simulink subsystem "Wind"  (R2025a)
settings: Solver=VariableStepAuto  StartTime=0.0  StopTime=10.0  RelTol=1e-3
model mask{windRating=0, maxWindSpeed=0, turbineOutput=0, frequency=0, windingRatio=0, rotorSpeed=0, windSpeed=0}
  mask prompts: windRating "Rating (kW)"; maxWindSpeed "Maximum Wind speed (m/s)"; turbineOutput "Turbine output (kW)"; frequency "Frequency (Hz)"; windingRatio "Transformer Ratio"; rotorSpeed "Rotor Speed (rpm)"; windSpeed "Wind Speed (m/s)"
libraries: fl_lib x19, ee_lib x8, nesl_utility x7
settings Model: DefaultTestHarness=Wind_Harness  Creator=skota  LastModifiedBy=skota

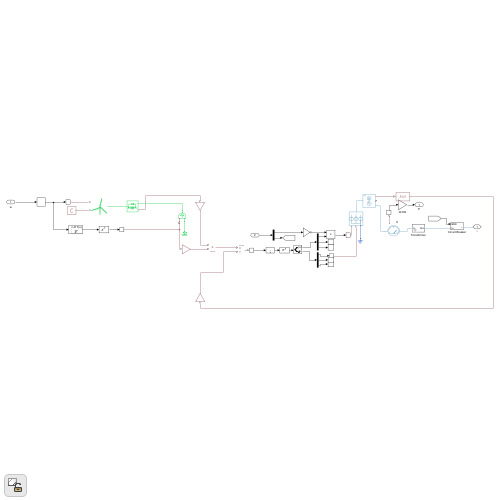
[thumbnail: Simulink's stored preview of the top-level diagram]
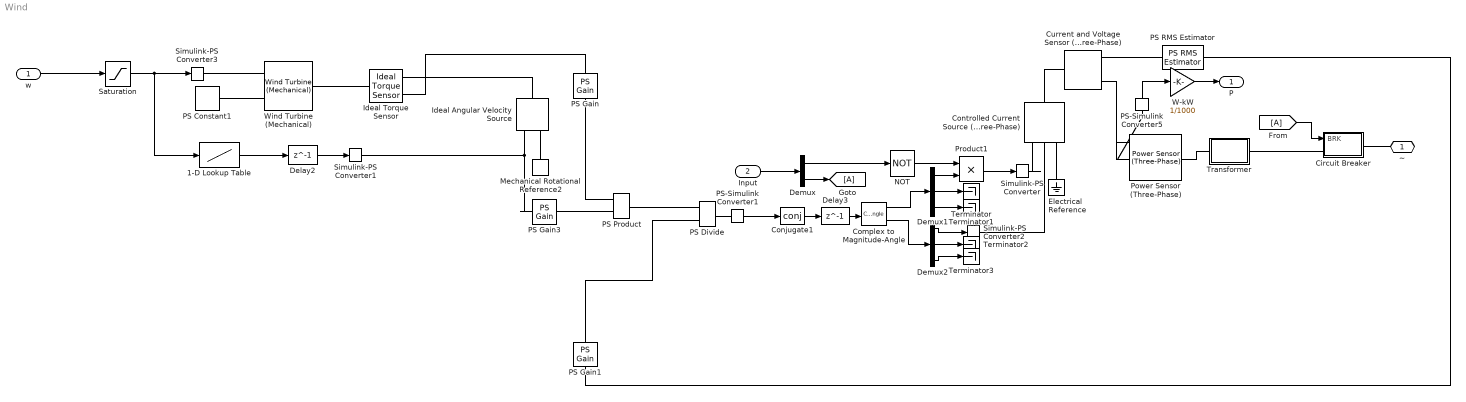
== system Wind ==
  w : Inport
  Input : Inport  Port=2
  1-D Lookup Table : Lookup_n-D  NumberOfTableDimensions=1  BreakpointsForDimension1=windSpeed  Table=rotorSpeed  InternalRulePriority=Speed  RndMeth=Simplest
  Circuit Breaker : Subsystem
  Complex to Magnitude-Angle : ComplexToMagnitudeAngle
  Conjugate1 : Math  Operator=conj  SignedPower=on  RndMeth=Zero
  Controlled Current Source (Three-Phase) : ee_lib/Sources/Controlled Current Source (Three-Phase)  input_option=ee.enum.inputType.singleFreqAC  FRated=frequency Hz
      settings: InternalSimscapePortConfiguration="{\"Bottom\":[],\"Left\":[{\"id\":\"It\",\"label\":\"I\",\"type\":\"input\"},{\"id\":\"ph\",\"label\":\"ph\",\"type\":\"input\"},{\"id\":\"n\",\"label\":\"n\",\"type\":\"foundation.electrical.electrical\"}],\"Right\":[{\"id\":\"N\",\"label\":\"~\",\"type\":\"foundation.electrical.three_phase\"}],\"Top\":[]}"
  Current and Voltage Sensor (Three-Phase) : ee_lib/Sensors & Transducers/Current and Voltage Sensor (Three-Phase)  vMeasurementType=ee.enum.vmeasurement.ll  outputUnit=ee.enum.unit.si  SRated=100e6 A*V  VRated=24e3 V  I_specify=off  I_priority=None  I=[0, 0, 0] A  I_nominal_specify=off  I_nominal_value=1  I_nominal_unit=A  V_specify=off  V_priority=None  V=[0, 0, 0] V  V_nominal_specify=off  V_nominal_value=1  V_nominal_unit=V
      settings: InternalSimscapePortConfiguration="{\"Bottom\":[],\"Left\":[{\"id\":\"N1\",\"label\":\"~1\",\"type\":\"foundation.electrical.three_phase\"}],\"Right\":[{\"id\":\"V_output\",\"label\":\"V\",\"type\":\"output\"},{\"id\":\"I_output\",\"label\":\"I\",\"type\":\"output\"},{\"id\":\"N2\",\"label\":\"~2\",\"type\":\"foundation.electrical.three_phase\"}],\"Top\":[]}"
  Delay2 : Delay  DelayLength=1  InitialCondition=1
  Delay3 : Delay  DelayLength=1  InitialCondition=1
  Demux : Demux  Outputs=2
  Demux1 : Demux  Outputs=3
  Demux2 : Demux  Outputs=3
  Electrical Reference : fl_lib/Electrical/Electrical Elements/Electrical Reference
  From : From
  Goto : Goto
  Ideal Angular Velocity Source : fl_lib/Mechanical/Mechanical Sources/Ideal Angular Velocity Source
  Ideal Torque Sensor : fl_lib/Mechanical/Mechanical Sensors/Ideal Torque Sensor
  Mechanical Rotational Reference2 : fl_lib/Mechanical/Rotational Elements/Mechanical Rotational Reference
  NOT : Logic  Operator=NOT  IconShape=distinctive  AllPortsSameDT=off  OutDataTypeStr=boolean
  PS Constant1 : fl_lib/Physical Signals/Sources/PS Constant  constant=0
  PS Divide : fl_lib/Physical Signals/Functions/PS Divide
  PS Gain : fl_lib/Physical Signals/Functions/PS Gain  gain=round(windRating/turbineOutput)
  PS Gain1 : fl_lib/Physical Signals/Functions/PS Gain  gain=sqrt(3)
  PS Gain3 : fl_lib/Physical Signals/Functions/PS Gain  gain=pi/30 rad/s
  PS Product : fl_lib/Physical Signals/Functions/PS Product
  PS RMS Estimator : fl_lib/Physical Signals/Periodic Operators/PS RMS Estimator  f0=frequency Hz
      settings: InternalSimscapePortConfiguration="{\"Bottom\":[],\"Left\":[{\"id\":\"I\",\"label\":\"\",\"type\":\"input\"}],\"Right\":[{\"id\":\"O\",\"label\":\"\",\"type\":\"output\"}],\"Top\":[]}"
  PS-Simulink Converter1 : nesl_utility/PS-Simulink Converter  PhysicalDomain=network_engine_domain  SubClassName=ps_output  LeftPortType=input  RightPortType=output  PseudoPeriodic=off  Frequencies=[]  VectorFormat=inherit  Unit=inherit  AffineConversion=off
  PS-Simulink Converter5 : nesl_utility/PS-Simulink Converter  PhysicalDomain=network_engine_domain  SubClassName=ps_output  LeftPortType=input  RightPortType=output  PseudoPeriodic=off  Frequencies=[]  VectorFormat=inherit  Unit=inherit  AffineConversion=off
  Power Sensor (Three-Phase) : ee_lib/Sensors & Transducers/Power Sensor (Three-Phase)  load_type=ee.enum.passive.type_balanced.balanced  f0=60 Hz  config=ee.enum.with_neutral.no  rho=1
      settings: InternalSimscapePortConfiguration="{\"Bottom\":[],\"Left\":[{\"id\":\"N1\",\"label\":\"~1\",\"type\":\"foundation.electrical.three_phase\"}],\"Right\":[{\"id\":\"N2\",\"label\":\"~2\",\"type\":\"foundation.electrical.three_phase\"}],\"Top\":[{\"id\":\"Pm\",\"label\":\"P\",\"type\":\"output\"},{\"id\":\"Qm\",\"label\":\"Q\",\"type\":\"output\"}]}"
  Product1 : Product
  Saturation : Saturate  UpperLimit=maxWindSpeed  LowerLimit=0
  Simulink-PS Converter : nesl_utility/Simulink-PS Converter  PhysicalDomain=network_engine_domain  SubClassName=ps_input  LeftPortType=input  RightPortType=output  PseudoPeriodic=off  Frequencies=[]  NoiseDistribution=none  NoiseParameters=[]  Unit=1  AffineConversion=off  FilteringAndDerivatives=provide  SimscapeFilterOrder=1  InputFilterTimeConstant=0.001  UdotUserProvided=0
  Simulink-PS Converter1 : nesl_utility/Simulink-PS Converter  PhysicalDomain=network_engine_domain  SubClassName=ps_input  LeftPortType=input  RightPortType=output  PseudoPeriodic=off  Frequencies=[]  NoiseDistribution=none  NoiseParameters=[]  Unit=rpm  AffineConversion=off  FilteringAndDerivatives=provide  SimscapeFilterOrder=1  InputFilterTimeConstant=0.001  UdotUserProvided=0
  Simulink-PS Converter2 : nesl_utility/Simulink-PS Converter  PhysicalDomain=network_engine_domain  SubClassName=ps_input  LeftPortType=input  RightPortType=output  PseudoPeriodic=off  Frequencies=[]  NoiseDistribution=none  NoiseParameters=[]  Unit=1  AffineConversion=off  FilteringAndDerivatives=provide  SimscapeFilterOrder=1  InputFilterTimeConstant=0.001  UdotUserProvided=0
  Simulink-PS Converter3 : nesl_utility/Simulink-PS Converter  PhysicalDomain=network_engine_domain  SubClassName=ps_input  LeftPortType=input  RightPortType=output  PseudoPeriodic=off  Frequencies=[]  NoiseDistribution=none  NoiseParameters=[]  Unit=m/s  AffineConversion=off  FilteringAndDerivatives=provide  SimscapeFilterOrder=1  InputFilterTimeConstant=0.001  UdotUserProvided=0
  Terminator{,1..3} (4 alike) : Terminator
  Transformer : Subsystem  mask{windingRatio=windingRatio}
      mask prompts: windingRatio "Winding ratio"
      mask DialogControl Container4 Prompt: General
  W-kW : Gain  Gain=1/1000
  Wind Turbine (Mechanical) : ee_lib/Electromechanical/Wind Turbine (Mechanical)  R_rotor=5.58 m  pitch_TLU=pitch deg  lambda_TLU=tsr  Cp_TLU=cp  v_thr=0.01 m/s  w_thr=0.01 rad/s  rho_air=1.225 kg/m^3  includeInertia=false  J=10e6 kg*m^2  lam=0 N*m*s/rad  w_specify=on  w_priority=None  w=0 rpm  w_nominal_specify=off  w_nominal_value=1  w_nominal_unit=rad/s  t_specify=off  t_priority=None  t=0 N*m  t_nominal_specify=off  t_nominal_value=1  t_nominal_unit=N*m  Torque_specify=off  Torque_priority=None  Torque=0 N*m  Torque_nominal_specify=off  Torque_nominal_value=1  Torque_nominal_unit=N*m
      settings: InternalSimscapePortConfiguration="{\"Bottom\":[],\"Left\":[{\"id\":\"vWind\",\"label\":\"V\",\"type\":\"input\"},{\"id\":\"pitch\",\"label\":\"β\",\"type\":\"input\"}],\"Right\":[{\"id\":\"R\",\"label\":\"R\",\"type\":\"foundation.mechanical.rotational.rotational\"}],\"Top\":[]}"
  ~ : PMIOPort  Side=Left
  P : Outport
  wires:
  Saturation/1 -> 1-D Lookup Table/1, Simulink-PS Converter3/1
  1-D Lookup Table/1 -> Delay2/1
  Demux2/1 -> Simulink-PS Converter2/1
  PS-Simulink Converter1/1 -> Conjugate1/1
  Delay3/1 -> Complex to Magnitude-Angle/1
  Delay2/1 -> Simulink-PS Converter1/1
  Conjugate1/1 -> Delay3/1
  Complex to Magnitude-Angle/1 -> Demux1/1
  Complex to Magnitude-Angle/2 -> Demux2/1
  PS-Simulink Converter5/1 -> W-kW/1
  From/1 -> Circuit Breaker/1(BRK)
  Demux1/1 -> Product1/2
  Product1/1 -> Simulink-PS Converter/1
  Demux/1 -> NOT/1
  NOT/1 -> Product1/1
  w/1 -> Saturation/1
  Demux1/2 -> Terminator/1
  Demux1/3 -> Terminator1/1
  Demux2/2 -> Terminator2/1
  Demux2/3 -> Terminator3/1
  W-kW/1 -> P/1
  Input/1 -> Demux/1
  Demux/2 -> Goto/1
  connections:
  PS Gain3/LConn1 -- Ideal Angular Velocity Source/RConn1 -- Simulink-PS Converter1/RConn1
  Ideal Torque Sensor/RConn1 -- Ideal Angular Velocity Source/LConn1
  PS Product/LConn1 -- PS Gain/RConn1
  PS Product/RConn1 -- PS Divide/LConn1
  PS Product/LConn2 -- PS Gain3/RConn1
  PS Gain/LConn1 -- Ideal Torque Sensor/RConn2
  PS-Simulink Converter1/LConn1 -- PS Divide/RConn1
  Electrical Reference/LConn1 -- Controlled Current Source (Three-Phase)/LConn3
  Power Sensor (Three-Phase)/LConn2 -- PS-Simulink Converter5/LConn1
  Simulink-PS Converter2/RConn1 -- Controlled Current Source (Three-Phase)/LConn2
  Current and Voltage Sensor (Three-Phase)/RConn3 -- Power Sensor (Three-Phase)/LConn1
  Current and Voltage Sensor (Three-Phase)/LConn1 -- Controlled Current Source (Three-Phase)/RConn1
  Wind Turbine (Mechanical)/LConn2 -- PS Constant1/RConn1
  Simulink-PS Converter/RConn1 -- Controlled Current Source (Three-Phase)/LConn1
  Wind Turbine (Mechanical)/LConn1 -- Simulink-PS Converter3/RConn1
  Ideal Torque Sensor/LConn1 -- Wind Turbine (Mechanical)/RConn1
  Mechanical Rotational Reference2/LConn1 -- Ideal Angular Velocity Source/RConn2
  Circuit Breaker/RConn1 -- ~/RConn1
  Current and Voltage Sensor (Three-Phase)/RConn1 -- PS RMS Estimator/LConn1
  PS RMS Estimator/RConn1 -- PS Gain1/LConn1
  PS Gain1/RConn1 -- PS Divide/LConn2
  Transformer/LConn1 -- Power Sensor (Three-Phase)/RConn1
  Transformer/RConn1 -- Circuit Breaker/LConn1

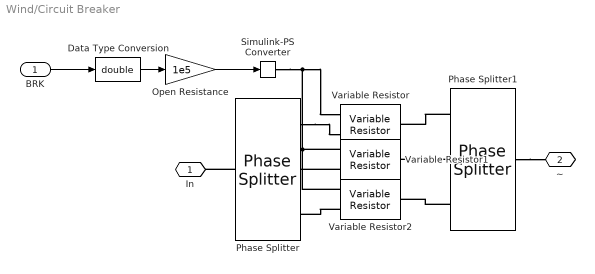
== system Wind/Circuit Breaker ==
  BRK : Inport
  Data Type Conversion : DataTypeConversion  OutDataTypeStr=double  SaturateOnIntegerOverflow=off  RndMeth=Floor
  Open Resistance : Gain  Gain=1e5
  Phase Splitter : ee_lib/Connectors & References/Phase Splitter
  Phase Splitter1 : ee_lib/Connectors & References/Phase Splitter
  Simulink-PS Converter : nesl_utility/Simulink-PS Converter  PhysicalDomain=network_engine_domain  SubClassName=ps_input  LeftPortType=input  RightPortType=output  PseudoPeriodic=off  Frequencies=[]  NoiseDistribution=none  NoiseParameters=[]  Unit=1  AffineConversion=off  FilteringAndDerivatives=provide  SimscapeFilterOrder=1  InputFilterTimeConstant=0.001  UdotUserProvided=0
  Variable Resistor : fl_lib/Electrical/Electrical Elements/Variable Resistor  Rmin=1e-4 Ohm  thermalEnable=false  thermal_mass=1 J/K  i_specify=off  i_priority=None  i=0 A  i_nominal_specify=off  i_nominal_value=1  i_nominal_unit=A  v_specify=off  v_priority=None  v=0 V  v_nominal_specify=off  v_nominal_value=1  v_nominal_unit=V  T_specify=off  T_priority=None  T=300 K  T_nominal_specify=off  T_nominal_value=1  T_nominal_unit=K
  Variable Resistor1 : fl_lib/Electrical/Electrical Elements/Variable Resistor  Rmin=1e-4 Ohm  thermalEnable=false  thermal_mass=1 J/K  i_specify=off  i_priority=None  i=0 A  i_nominal_specify=off  i_nominal_value=1  i_nominal_unit=A  v_specify=off  v_priority=None  v=0 V  v_nominal_specify=off  v_nominal_value=1  v_nominal_unit=V  T_specify=off  T_priority=None  T=300 K  T_nominal_specify=off  T_nominal_value=1  T_nominal_unit=K
  Variable Resistor2 : fl_lib/Electrical/Electrical Elements/Variable Resistor  Rmin=1e-4 Ohm  thermalEnable=false  thermal_mass=1 J/K  i_specify=off  i_priority=None  i=0 A  i_nominal_specify=off  i_nominal_value=1  i_nominal_unit=A  v_specify=off  v_priority=None  v=0 V  v_nominal_specify=off  v_nominal_value=1  v_nominal_unit=V  T_specify=off  T_priority=None  T=300 K  T_nominal_specify=off  T_nominal_value=1  T_nominal_unit=K
  In : PMIOPort  Side=Left
  ~ : PMIOPort  Port=2  Side=Right
  wires:
  Open Resistance/1 -> Simulink-PS Converter/1
  BRK/1 -> Data Type Conversion/1
  Data Type Conversion/1 -> Open Resistance/1
  connections:
  Phase Splitter/LConn1 -- In/RConn1
  Variable Resistor1/LConn1 -- Variable Resistor2/LConn1 -- Simulink-PS Converter/RConn1 -- Variable Resistor/LConn1
  Phase Splitter1/LConn1 -- ~/RConn1
  Phase Splitter1/RConn1 -- Variable Resistor/RConn1
  Variable Resistor2/LConn2 -- Phase Splitter/RConn3
  Phase Splitter/RConn1 -- Variable Resistor/LConn2
  Phase Splitter1/RConn3 -- Variable Resistor2/RConn1
  Variable Resistor1/LConn2 -- Phase Splitter/RConn2
  Phase Splitter1/RConn2 -- Variable Resistor1/RConn1

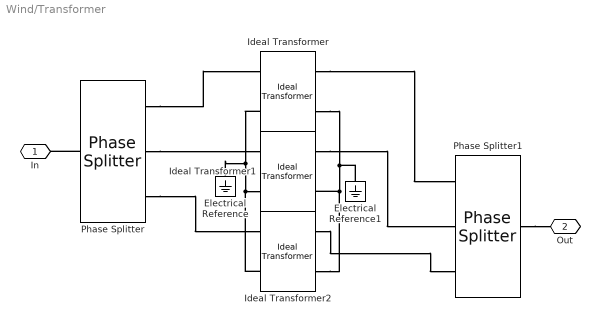
== system Wind/Transformer ==
  Electrical Reference : fl_lib/Electrical/Electrical Elements/Electrical Reference
  Electrical Reference1 : fl_lib/Electrical/Electrical Elements/Electrical Reference
  Ideal Transformer : fl_lib/Electrical/Electrical Elements/Ideal Transformer  n=windingRatio  i1_specify=off  i1_priority=None  i1=0 A  i1_nominal_specify=off  i1_nominal_value=1  i1_nominal_unit=A  v1_specify=off  v1_priority=None  v1=0 V  v1_nominal_specify=off  v1_nominal_value=1  v1_nominal_unit=V  i2_specify=off  i2_priority=None  i2=0 A  i2_nominal_specify=off  i2_nominal_value=1  i2_nominal_unit=A  v2_specify=off  v2_priority=None  v2=0 V  v2_nominal_specify=off  v2_nominal_value=1  v2_nominal_unit=V
  Ideal Transformer1 : fl_lib/Electrical/Electrical Elements/Ideal Transformer  n=windingRatio  i1_specify=off  i1_priority=None  i1=0 A  i1_nominal_specify=off  i1_nominal_value=1  i1_nominal_unit=A  v1_specify=off  v1_priority=None  v1=0 V  v1_nominal_specify=off  v1_nominal_value=1  v1_nominal_unit=V  i2_specify=off  i2_priority=None  i2=0 A  i2_nominal_specify=off  i2_nominal_value=1  i2_nominal_unit=A  v2_specify=off  v2_priority=None  v2=0 V  v2_nominal_specify=off  v2_nominal_value=1  v2_nominal_unit=V
  Ideal Transformer2 : fl_lib/Electrical/Electrical Elements/Ideal Transformer  n=windingRatio  i1_specify=off  i1_priority=None  i1=0 A  i1_nominal_specify=off  i1_nominal_value=1  i1_nominal_unit=A  v1_specify=off  v1_priority=None  v1=0 V  v1_nominal_specify=off  v1_nominal_value=1  v1_nominal_unit=V  i2_specify=off  i2_priority=None  i2=0 A  i2_nominal_specify=off  i2_nominal_value=1  i2_nominal_unit=A  v2_specify=off  v2_priority=None  v2=0 V  v2_nominal_specify=off  v2_nominal_value=1  v2_nominal_unit=V
  Phase Splitter : ee_lib/Connectors & References/Phase Splitter
  Phase Splitter1 : ee_lib/Connectors & References/Phase Splitter
  In : PMIOPort  Side=Left
  Out : PMIOPort  Port=2  Side=Right
  connections:
  Ideal Transformer/RConn2 -- Electrical Reference1/LConn1 -- Ideal Transformer1/RConn2 -- Ideal Transformer2/RConn2
  Phase Splitter/RConn3 -- Ideal Transformer2/LConn1
  Phase Splitter/RConn2 -- Ideal Transformer1/LConn1
  Phase Splitter/RConn1 -- Ideal Transformer/LConn1
  Ideal Transformer/LConn2 -- Electrical Reference/LConn1 -- Ideal Transformer1/LConn2 -- Ideal Transformer2/LConn2
  Phase Splitter/LConn1 -- In/RConn1
  Phase Splitter1/LConn1 -- Out/RConn1
  Ideal Transformer/RConn1 -- Phase Splitter1/RConn1
  Ideal Transformer2/RConn1 -- Phase Splitter1/RConn3
  Ideal Transformer1/RConn1 -- Phase Splitter1/RConn2
